simulink model "robotModel_blackbox"  (R2023a)
settings: Solver=FixedStepAuto  StartTime=0.0  StopTime=0.1  RelTol=1e-3
values from neighbouring files (symbols this model uses):
  theta1 = theta1_test(i)    [getSimData-1.m]
  theta2 = theta2_test(i)    [getSimData-1.m]
settings Model: Creator=tuanwin11  LastModifiedBy=tuanwin11

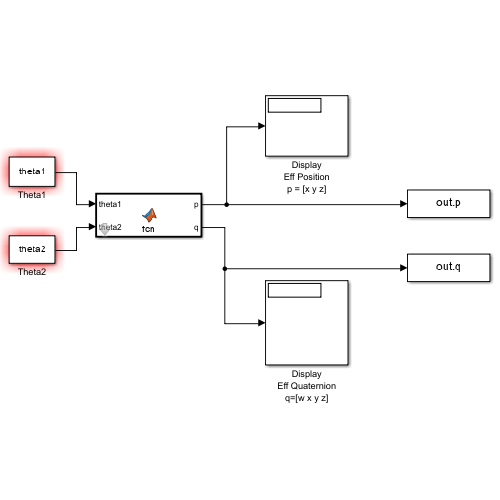
[thumbnail: Simulink's stored preview of the top-level diagram]
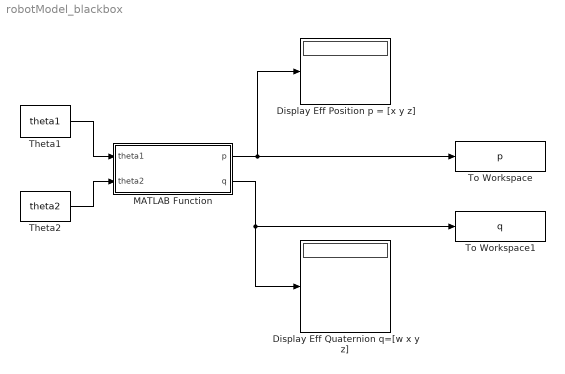
== system robotModel_blackbox ==
  Display Eff Position p = [x y z] : Display
  Display Eff Quaternion q=[w x y z] : Display
  MATLAB Function : MATLAB Function  TreatAsAtomicUnit=on
  "Theta1 " : Constant  Value=theta1
  "Theta2 " : Constant  Value=theta2
  To Workspace : ToWorkspace  VariableName=p  SaveFormat=Timeseries  SampleTime=-1
  To Workspace1 : ToWorkspace  VariableName=q  SaveFormat=Timeseries  SampleTime=-1
  wires:
  "Theta1 "/1 -> MATLAB Function/1(theta1)
  "Theta2 "/1 -> MATLAB Function/2(theta2)
  MATLAB Function/1(p) -> To Workspace/1, Display Eff Position p = [x y z]/1
  MATLAB Function/2(q) -> To Workspace1/1, Display Eff Quaternion q=[w x y z]/1

== matlab function robotModel_blackbox/MATLAB Function ==
  data: theta1 input; p output; theta2 input; q output
function [p, q] = fcn(theta1, theta2)
% Nominal parameters
d1N = 0; theta1N = theta1;  a1N = 0.1;  alpha1N = 0;
d2N = 0; theta2N = theta2; a2N = 0.2;  alpha2N = 0;

% Errors
% theta
detltaTheta1 = 0.1; deltaTheta2 = 0.1;
% d
deltaD1 = 0.01;
deltaD2 = 0.03;
% a
deltaA1 = 0.05; deltaA2 = 0.05;
% alpha
deltaAlpha1 = 0.2;
deltaAlpha2 = 0.0;

% Real paramters
% link 1
d1 = d1N + deltaD1;
theta1 = theta1N + detltaTheta1;
a1 = a1N + deltaA1;
alpha1 = alpha1N + deltaAlpha1;

% link 2
d2 = d2N + deltaD2;
theta2 = theta2N + deltaTheta2;
a2 = a2N + deltaA2;
alpha2 = alpha2N + deltaAlpha2;

T10 = DH_mat([d1, theta1, a1, alpha1]); 
T21 = DH_mat([d2, theta2, a2, alpha2]); 

%T10 = Rotz(theta1)*Trans_d(d1)*Trans_a(a1)*Rotx(alpha1);
%T21 = Rotz(theta2)*Trans_d(d2)*Trans_a(a2)*Rotx(alpha2);

T_eff = T10*T21;

% end effector position
p = T_eff(1:3, 4);
% end effector quaternion
R = T_eff(1:3, 1:3);
q = rotm2quat(R);

end

function T = DH_mat(x)
d = x(1);
theta = x(2);
a = x(3);
alpha = x(4);

T = zeros(4,4);
T(4,4) = 1;

T(1,1) = cos(theta);    T(1,2) = -sin(theta)*cos(alpha);    T(1,3) = sin(theta)*sin(alpha); T(1,4) = a*cos(theta);
T(2,1) = sin(theta);    T(2,2) = cos(theta)*cos(alpha); T(2,3) = -cos(theta)*sin(alpha);    T(2,4) = a*sin(theta);
T(3,2) = sin(alpha);    T(3,3) = cos(alpha);    T(3,4) = d;

end


function y = Rotz(theta)

y = [cos(theta) -sin(theta) 0 0;...
          sin(theta)  cos(theta) 0 0;...
          0 0 1 0;...
          0 0 0 1];
end

function y = Trans_d(d)
y = [1 0 0 0;...
     0 1 0 0;...
     0 0 1 d;...
     0 0 0 1];
end
function y = Trans_a(a)
y = [1 0 0 a;...
     0 1 0 0;...
     0 0 1 0;...
     0 0 0 1];
end
function y = Rotx(alpha)
y = [1 0 0 0;...
     0 cos(alpha) -sin(alpha) 0;...
     0 sin(alpha) cos(alpha) 0;...
     0 0 0 1];
end
